simulink model "network2"  (R2023a)
settings: Solver=VariableStepAuto  StartTime=0.0  StopTime=inf  RelTol=1e-3
InitFcn:
  | model_init
values from neighbouring files (symbols this model uses):
  F0 = 1800    [model_init.m]
  Tb = 1/1200    (= 0.000833333333333)    [model_init.m]
  Ts = Tb/8    (= 0.000104166666667)    [model_init.m]
libraries: dspsrcs4 x2, commsink2 x1, commchan3 x1, commrandsrc3 x1, hdlsllib x1, commfilt2 x1
settings Model: Creator=mfera  LastModifiedBy=vadim
settings ModelReferenceCC: EnableRefExpFcnMdlSchedulingChecks=on

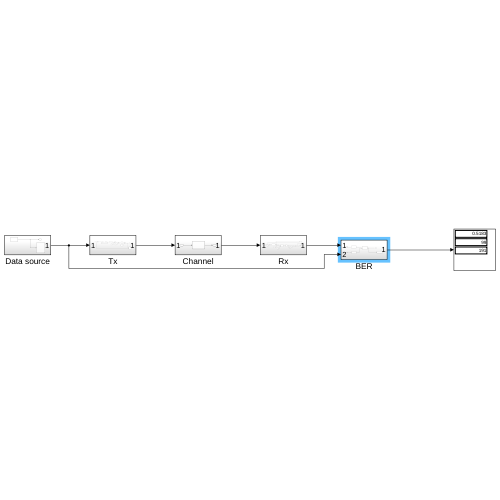
[thumbnail: Simulink's stored preview of the top-level diagram]
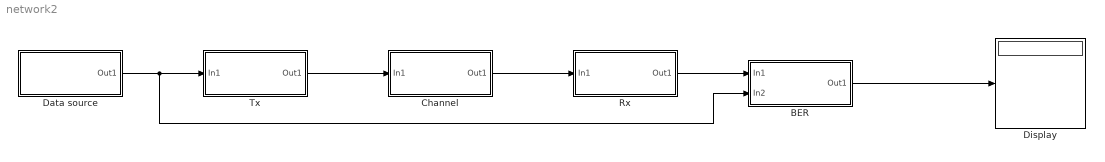
== system network2 ==
  BER : Subsystem
  Channel : Subsystem
  Data source : Subsystem
  Display : Display
      settings: Decimation=3
  Rx : Subsystem
  Tx : Subsystem
  wires:
  Data source/1(Out1) -> BER/2(In2), Tx/1(In1)
  Tx/1(Out1) -> Channel/1(In1)
  Channel/1(Out1) -> Rx/1(In1)
  Rx/1(Out1) -> BER/1(In1)
  BER/1(Out1) -> Display/1

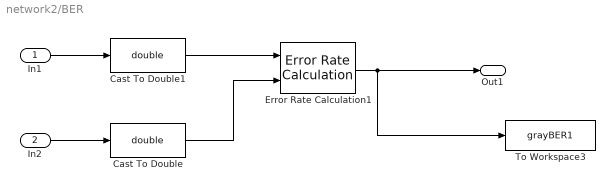
== system network2/BER ==
  In1 : Inport
  In2 : Inport  Port=2
  Cast To Double : DataTypeConversion  OutDataTypeStr=double  SaturateOnIntegerOverflow=off  RndMeth=Floor
  Cast To Double1 : DataTypeConversion  OutDataTypeStr=double  SaturateOnIntegerOverflow=off  RndMeth=Floor
  Error Rate Calculation1 : commsink2/Error Rate Calculation  N=1  st_delay=0  cp_mode=Entire frame  subframe=[]  PMode=Port  WsName=ErrorVec  RsMode2=off  stop=on  numErr=100  maxBits=1e8
  To Workspace3 : ToWorkspace  VariableName=grayBER1  SampleTime=-1
      settings: Save2DSignal=2-D array (concatenate along first dimension)
  Out1 : Outport
  wires:
  In1/1 -> Cast To Double1/1
  In2/1 -> Cast To Double/1
  Cast To Double1/1 -> Error Rate Calculation1/1
  Cast To Double/1 -> Error Rate Calculation1/2
  Error Rate Calculation1/1 -> To Workspace3/1, Out1/1

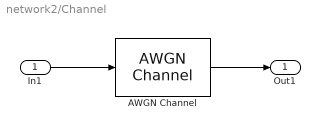
== system network2/Channel ==
  In1 : Inport
  AWGN Channel : commchan3/AWGN Channel  LegacyMode=on  NoiseMethod="Signal to noise ratio  (SNR)"  noiseMode="Signal to noise ratio  (Eb/No)"  EbNo=10  EsNo=10  SNR=10  BitsPerSymbol=1  SignalPower=0.5  SamplesPerSymbol=1  SymbolPeriod=Tb  VarianceSource=Parameter  Variance=1  RandomStream=Global stream  Seed=67  SimulateUsing=Code generation
  Out1 : Outport
  wires:
  In1/1 -> AWGN Channel/1
  AWGN Channel/1 -> Out1/1

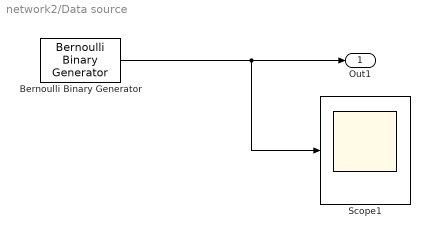
== system network2/Data source ==
  Bernoulli Binary Generator : commrandsrc3/Bernoulli Binary Generator  ProbabilityOfZero=0.5  SeedSource=Auto  Seed=0  SampleTime=Tb  SamplesPerFrame=1  OutputDataType=double  SimulateUsing=Interpreted execution
  Scope1 : Scope
  Out1 : Outport
  wires:
  Bernoulli Binary Generator/1 -> Scope1/1, Out1/1

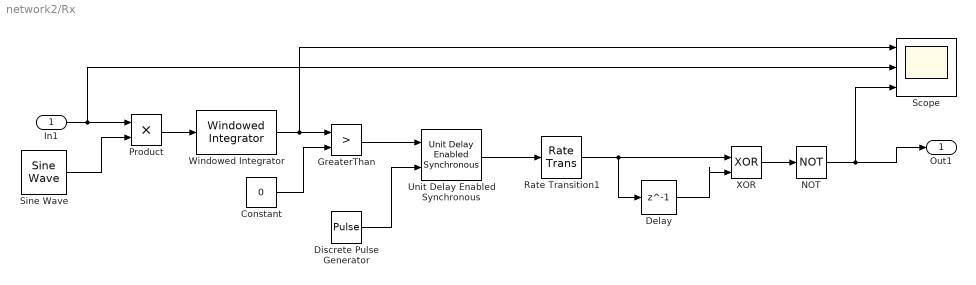
== system network2/Rx ==
  In1 : Inport
  Constant : Constant  Value=0
  Delay : Delay  DelayLength=1  InitialCondition=0
  Discrete Pulse Generator : DiscretePulseGenerator  Period=Tb/Ts  PhaseDelay=Tb/Ts-1  SampleTime=Ts
  GreaterThan : RelationalOperator  Operator=>  OutDataTypeStr=boolean  RndMeth=Simplest  InputSameDT=off
  NOT : Logic  Operator=NOT  IconShape=distinctive  AllPortsSameDT=off  OutDataTypeStr=boolean
  Product : Product
  Rate Transition1 : RateTransition  OutPortSampleTime=Tb
  Scope : Scope  NumInputPorts=3
  Sine Wave : dspsrcs4/Sine Wave  Amplitude=1  Frequency=F0  Phase=0  SampleMode=Discrete  OutComplex=Real  CompMethod=Trigonometric fcn  TableSize=Speed  SampleTime=Ts  SamplesPerFrame=1  ResetState=Restart at time zero  OutputFrames=off  dataType=double  wordLen=16  udDataType=sfix(16)  fracBitsMode=Best precision  numFracBits=15  OutDataTypeStr=double  LastOutDataTypeStr=double
  Unit Delay Enabled Synchronous : hdlsllib/Discrete/Unit Delay Enabled Synchronous  InitialCondition=0.0  SampleTime=-1
  Windowed Integrator : commfilt2/Windowed Integrator  integperiod=Tb/Ts  InputProcessing=Columns as channels (frame based)  roundingMode=Floor  overflowMode=off  coeffDataTypeStr=Inherit: Same word length as input  coeffMin=[]  coeffMax=[]  coeffLastDataTypeStr=Inherit: Same word length as input  accumDataTypeStr=Inherit: Same as product output  accumLastDataTypeStr=Inherit: Same as product output  outputDataTypeStr=Inherit: Same as accumulator  outputMin=[]  outputMax=[]  outputLastDataTypeStr=Inherit: Same as accumulator
  XOR : Logic  Operator=XOR  IconShape=distinctive  AllPortsSameDT=off  OutDataTypeStr=boolean
  Out1 : Outport
  wires:
  In1/1 -> Scope/2, Product/1
  Sine Wave/1 -> Product/2
  Product/1 -> Windowed Integrator/1
  Windowed Integrator/1 -> Scope/1, GreaterThan/1
  Constant/1 -> GreaterThan/2
  XOR/1 -> NOT/1
  NOT/1 -> Scope/3, Out1/1
  Rate Transition1/1 -> XOR/1, Delay/1
  Delay/1 -> XOR/2
  GreaterThan/1 -> Unit Delay Enabled Synchronous/1
  Discrete Pulse Generator/1 -> Unit Delay Enabled Synchronous/2
  Unit Delay Enabled Synchronous/1 -> Rate Transition1/1

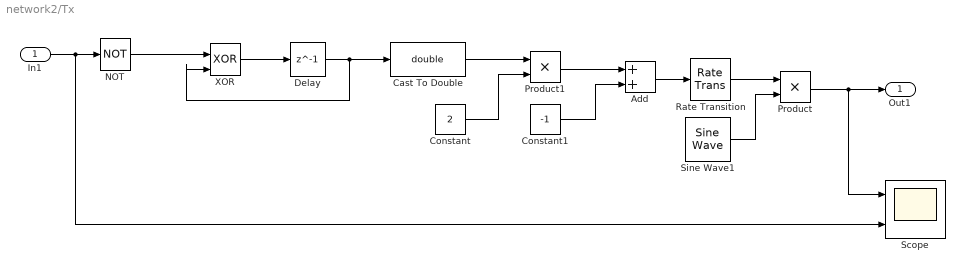
== system network2/Tx ==
  In1 : Inport
  Add : Sum
  Cast To Double : DataTypeConversion  OutDataTypeStr=double  SaturateOnIntegerOverflow=off  RndMeth=Floor
  Constant : Constant  Value=2
  Constant1 : Constant  Value=-1
  Delay : Delay  DelayLength=1  InitialCondition=0
  NOT : Logic  Operator=NOT  IconShape=distinctive  AllPortsSameDT=off  OutDataTypeStr=boolean
  Product : Product
  Product1 : Product
  Rate Transition : RateTransition
  Scope : Scope  NumInputPorts=2
  Sine Wave1 : dspsrcs4/Sine Wave  Amplitude=1  Frequency=F0  Phase=0  SampleMode=Discrete  OutComplex=Real  CompMethod=Trigonometric fcn  TableSize=Speed  SampleTime=Ts  SamplesPerFrame=1  ResetState=Restart at time zero  OutputFrames=off  dataType=double  wordLen=16  udDataType=sfix(16)  fracBitsMode=Best precision  numFracBits=15  OutDataTypeStr=double  LastOutDataTypeStr=double
  XOR : Logic  Operator=XOR  IconShape=distinctive  AllPortsSameDT=off  OutDataTypeStr=boolean
  Out1 : Outport
  wires:
  In1/1 -> Scope/2, NOT/1
  NOT/1 -> XOR/1
  XOR/1 -> Delay/1
  Delay/1 -> Cast To Double/1, XOR/2
  Cast To Double/1 -> Product1/1
  Constant/1 -> Product1/2
  Product1/1 -> Add/1
  Constant1/1 -> Add/2
  Add/1 -> Rate Transition/1
  Sine Wave1/1 -> Product/2
  Rate Transition/1 -> Product/1
  Product/1 -> Scope/1, Out1/1
